simulink model "IO601canmultiplemessageloopback"  (R2013a)
settings: Solver=FixedStepDiscrete  StartTime=0.0  StopTime=inf  RelTol=1e-3
libraries: canmsglib x5, dspmtrx3 x5, speedgoatlib_IO601 x3, xpclib x3
Description:
  | 7.14.0.739 (R2012a)
settings Model: BufferReuse=off  Creator=cedric  LastModifiedBy=lab3
settings SolverCC: EnableConcurrentExecution=on
settings DataIOCC: SignalLoggingSaveFormat=ModelDataLogs
settings OptimizationCC: BlockReduction=off  BooleanDataType=off  OptimizeBlockIOStorage=off  BufferReuse=off  ExpressionFolding=off  ExpressionDepthLimit=2147483647  LocalBlockOutputs=off
settings DebuggingCC: FcnCallInpInsideContextMsg=UseLocalSettings
settings HardwareCC: ProdIntDivRoundTo=Zero  ProdEndianess=LittleEndian  ProdHWDeviceType=Generic->32-bit x86 compatible
settings RTWCC: SystemTargetFile=xpctarget.tlc  TemplateMakefile=xpc_default_tmf  Description=Simulink Real-Time  RTWVerbose=off  ProcessScript=xpctarget_make_rtw_hook  RTWCompilerOptimization=On
settings xpcTargetCC: TargetFcnLib=ansi_tfl_table_tmw.mat  CodeReplacementLibrary=XPC_BLAS  ParMdlRefBuildCompliant=on  ConcurrentExecutionCompliant=on  CombineSignalStateStructs=off  MATLABClassNameForMDSCustomization=xpcAperiodicCustomization  GRTInterface=on  GenerateAllocFcn=off  xPCTaskExecutionProfile=off  xPCRL32EventNumber=5000  xPCLoadParamSetFile=off  xPCConcurrentTasks=off  xPCEnableSFAnimation=off

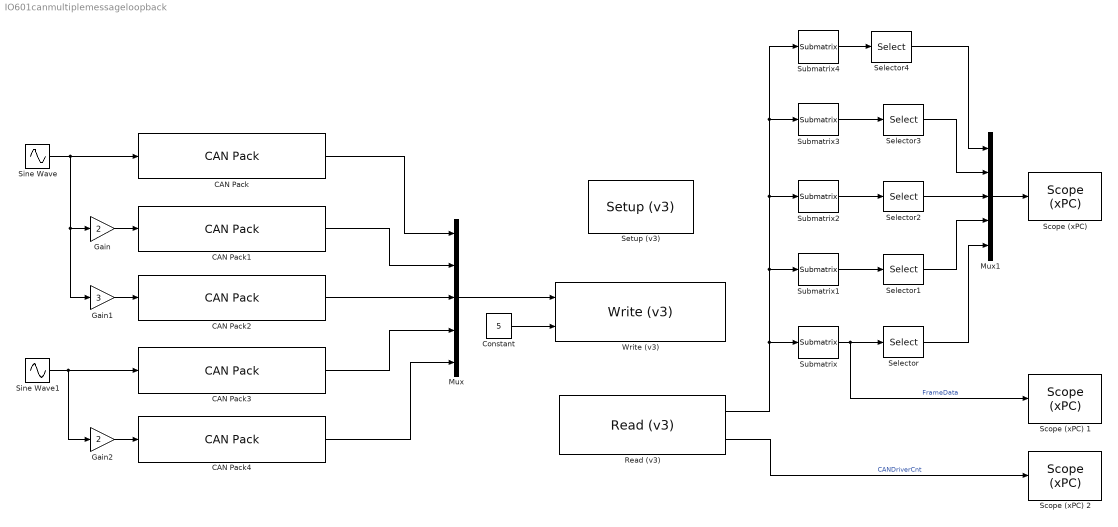
== system IO601canmultiplemessageloopback ==
  CAN Pack : canmsglib/CAN Pack  MsgList=(none)  MsgName=Test message  MsgIDType=Extended (29-bit identifier)  MsgIdentifier=1048575  MsgLength=8  SignalInfo=Signal1$0$64$1$4$1$0$1$0$-Inf$Inf$#  NSignals=1  StartBits=str2num('[int32(0)]')  SignalSizes=str2num('[int32(64)]')  ByteOrders=str2num('[int32(1)]')  DataTypes=str2num('[int32(4)]')  MultiplexTypes=str2num('[int32(1)]')  MultiplexValues=str2num('[double(0)]')  Factors=str2num('[double(1)]')  Offsets=str2num('[double(0)]')  Minimums=str2num('[double(-Inf)]')  Maximums=str2num('[double(Inf)]')  Remote=off
      settings: DataFormat=manually specified signals
  CAN Pack1 : canmsglib/CAN Pack  MsgList=(none)  MsgName=Test message  MsgIDType=Extended (29-bit identifier)  MsgIdentifier=1048575  MsgLength=8  SignalInfo=Signal1$0$64$1$4$1$0$1$0$-Inf$Inf$#  NSignals=1  StartBits=str2num('[int32(0)]')  SignalSizes=str2num('[int32(64)]')  ByteOrders=str2num('[int32(1)]')  DataTypes=str2num('[int32(4)]')  MultiplexTypes=str2num('[int32(1)]')  MultiplexValues=str2num('[double(0)]')  Factors=str2num('[double(1)]')  Offsets=str2num('[double(0)]')  Minimums=str2num('[double(-Inf)]')  Maximums=str2num('[double(Inf)]')  Remote=off
      settings: DataFormat=manually specified signals
  CAN Pack2 : canmsglib/CAN Pack  MsgList=(none)  MsgName=Test message  MsgIDType=Extended (29-bit identifier)  MsgIdentifier=1048575  MsgLength=8  SignalInfo=Signal1$0$64$1$4$1$0$1$0$-Inf$Inf$#  NSignals=1  StartBits=str2num('[int32(0)]')  SignalSizes=str2num('[int32(64)]')  ByteOrders=str2num('[int32(1)]')  DataTypes=str2num('[int32(4)]')  MultiplexTypes=str2num('[int32(1)]')  MultiplexValues=str2num('[double(0)]')  Factors=str2num('[double(1)]')  Offsets=str2num('[double(0)]')  Minimums=str2num('[double(-Inf)]')  Maximums=str2num('[double(Inf)]')  Remote=off
      settings: DataFormat=manually specified signals
  CAN Pack3 : canmsglib/CAN Pack  MsgList=(none)  MsgName=Test message  MsgIDType=Extended (29-bit identifier)  MsgIdentifier=2000  MsgLength=8  SignalInfo=Signal1$0$64$1$4$1$0$1$0$-Inf$Inf$#  NSignals=1  StartBits=str2num('[int32(0)]')  SignalSizes=str2num('[int32(64)]')  ByteOrders=str2num('[int32(1)]')  DataTypes=str2num('[int32(4)]')  MultiplexTypes=str2num('[int32(1)]')  MultiplexValues=str2num('[double(0)]')  Factors=str2num('[double(1)]')  Offsets=str2num('[double(0)]')  Minimums=str2num('[double(-Inf)]')  Maximums=str2num('[double(Inf)]')  Remote=off
      settings: DataFormat=manually specified signals
  CAN Pack4 : canmsglib/CAN Pack  MsgList=(none)  MsgName=Test message  MsgIDType=Extended (29-bit identifier)  MsgIdentifier=2000  MsgLength=8  SignalInfo=Signal1$0$64$1$4$1$0$1$0$-Inf$Inf$#  NSignals=1  StartBits=str2num('[int32(0)]')  SignalSizes=str2num('[int32(64)]')  ByteOrders=str2num('[int32(1)]')  DataTypes=str2num('[int32(4)]')  MultiplexTypes=str2num('[int32(1)]')  MultiplexValues=str2num('[double(0)]')  Factors=str2num('[double(1)]')  Offsets=str2num('[double(0)]')  Minimums=str2num('[double(-Inf)]')  Maximums=str2num('[double(Inf)]')  Remote=off
      settings: DataFormat=manually specified signals
  Constant : Constant  Value=5
  Gain : Gain  Gain=2
  Gain1 : Gain  Gain=3
  Gain2 : Gain  Gain=2
  Mux : Mux  Inputs=5
  Mux1 : Mux  Inputs=5
  Read (v3) : speedgoatlib_IO601/Read (v3)  id=1  outputFormat=Matrix of doubles (legacy)  port1=off  port2=on  depth1=10  depth2=5  sampletime=0.005  pciSlot=-1
  Scope (xPC) : xpclib/Misc./Scope (xPC)   scopeno=1  scopetype=Target  autostart=on  viewmode=Graphical redraw  formatstr='%15.6f'  grid=on  ylimits=[0,0]  nosamples=250  noprepostsamples=0  interleave=1  triggermode=Signal triggering  triggersignal=5  trigsignalfromport=off  triggerlevel=0.5  triggerslope=Rising  triggerscope=1  triggersample=0  filename=data.dat  mode=Lazy  writesize=512  autorestart=off  dynamicfilemode=off  maxwritefilesize=512*1024^2
  Scope (xPC) 1 : xpclib/Misc./Scope (xPC)   scopeno=2  scopetype=Target  autostart=on  viewmode=Numerical  formatstr='%15.6f'  grid=on  ylimits=[0,0]  nosamples=3  noprepostsamples=0  interleave=1  triggermode=FreeRun  triggersignal=1  trigsignalfromport=off  triggerlevel=0.0  triggerslope=Rising  triggerscope=1  triggersample=0  filename=data.dat  mode=Lazy  writesize=512  autorestart=off  dynamicfilemode=off  maxwritefilesize=512*1024^2
  Scope (xPC) 2 : xpclib/Misc./Scope (xPC)   scopeno=3  scopetype=Target  autostart=on  viewmode=Numerical  formatstr='%15.6f'  grid=on  ylimits=[0,0]  nosamples=3  noprepostsamples=0  interleave=1  triggermode=FreeRun  triggersignal=1  trigsignalfromport=off  triggerlevel=0.0  triggerslope=Rising  triggerscope=1  triggersample=0  filename=data.dat  mode=Lazy  writesize=512  autorestart=off  dynamicfilemode=off  maxwritefilesize=512*1024^2
  Selector{,1..4} (5 alike) : Selector  InputPortWidth=6  Indices=[6]
  Setup (v3) : speedgoatlib_IO601/Setup (v3)  id=1  can1enable=on  can1bus=Highspeed  can1Baudrate=1 MBaud  can1UserBR=[1,1,5,2]  stdAcc1=[0,0,0,0]  extAcc1=[0,0,0,0]  can2enable=on  can2bus=Highspeed  can2Baudrate=1 MBaud  can2UserBR=[1,1,5,2]  stdAcc2=[0,0,0,0]  extAcc2=[double(hex2dec('1FFFFFFF')), 2000, double(hex2dec('1FFFFFFF')), 1048575]  pciSlot=-1
  Sine Wave : Sin  Amplitude=10  Frequency=2*pi*10  Samples=100
  Sine Wave1 : Sin  Amplitude=10  Frequency=2*pi*5  Samples=100
  Submatrix : dspmtrx3/Submatrix  RowSpan=One row  RowStartMode=Index  RowStartIndex=1  RowEndMode=Last  RowEndIndex=1  ColSpan=All columns  ColStartMode=First  ColStartIndex=1  ColEndMode=Last  ColEndIndex=1
  Submatrix1 : dspmtrx3/Submatrix  RowSpan=One row  RowStartMode=Index  RowStartIndex=2  RowEndMode=Last  RowEndIndex=1  ColSpan=All columns  ColStartMode=First  ColStartIndex=1  ColEndMode=Last  ColEndIndex=1
  Submatrix2 : dspmtrx3/Submatrix  RowSpan=One row  RowStartMode=Index  RowStartIndex=3  RowEndMode=Last  RowEndIndex=1  ColSpan=All columns  ColStartMode=First  ColStartIndex=1  ColEndMode=Last  ColEndIndex=1
  Submatrix3 : dspmtrx3/Submatrix  RowSpan=One row  RowStartMode=Index  RowStartIndex=4  RowEndMode=Last  RowEndIndex=1  ColSpan=All columns  ColStartMode=First  ColStartIndex=1  ColEndMode=Last  ColEndIndex=1
  Submatrix4 : dspmtrx3/Submatrix  RowSpan=One row  RowStartMode=Index  RowStartIndex=5  RowEndMode=Last  RowEndIndex=1  ColSpan=All columns  ColStartMode=First  ColStartIndex=1  ColEndMode=Last  ColEndIndex=1
  Write (v3) : speedgoatlib_IO601/Write (v3)  Priority=1  id=1  sampletime=0.005  pciSlot=-1  inputType=CAN_MESSAGE plus count  port=1  maxMsg=5  status=off  init=[]  term=[]
  wires:
  Constant/1 -> Write (v3)/2
  Read (v3)/1 -> Submatrix/1, Submatrix1/1, Submatrix2/1, Submatrix3/1, Submatrix4/1
  CAN Pack1/1 -> Mux/2
  Sine Wave/1 -> Gain1/1, Gain/1, CAN Pack/1
  CAN Pack/1 -> Mux/1
  Mux/1 -> Write (v3)/1
  CAN Pack2/1 -> Mux/3
  CAN Pack3/1 -> Mux/4
  CAN Pack4/1 -> Mux/5
  Read (v3)/2 -> Scope (xPC) 2/1  "CANDriverCnt"
  Submatrix/1 -> Selector/1, Scope (xPC) 1/1  "FrameData"
  Selector/1 -> Mux1/5
  Sine Wave1/1 -> Gain2/1, CAN Pack3/1
  Submatrix4/1 -> Selector4/1
  Selector4/1 -> Mux1/1
  Selector3/1 -> Mux1/2
  Submatrix3/1 -> Selector3/1
  Submatrix2/1 -> Selector2/1
  Selector2/1 -> Mux1/3
  Selector1/1 -> Mux1/4
  Mux1/1 -> Scope (xPC)/1
  Submatrix1/1 -> Selector1/1
  Gain/1 -> CAN Pack1/1
  Gain1/1 -> CAN Pack2/1
  Gain2/1 -> CAN Pack4/1
